simulink model "lab01"  (R2018a)
settings: Solver=VariableStepAuto  StartTime=0.0  StopTime=10.0  RelTol=1e-3
values from neighbouring files (symbols this model uses):
  dt = 5e-3    (= 0.005)    [lab0.m]    (also in lab0_step.m)
libraries: legoev3lib x4
settings Model: Creator=jacobdelrosario  LastModifiedBy=jacobdelrosario

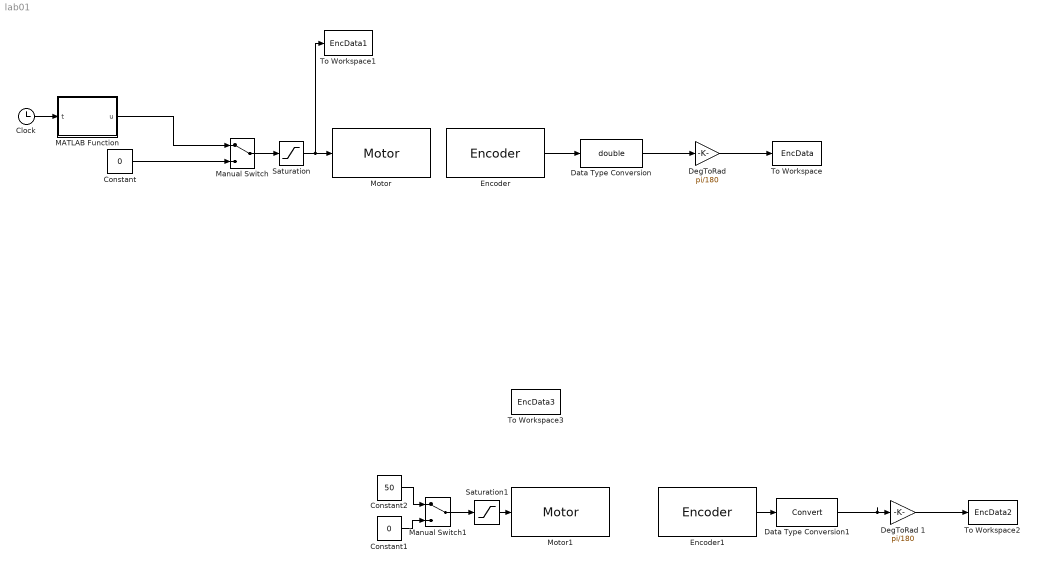
== system lab01 ==
  Clock : Clock
  Constant : Constant  Value=0  SampleTime=dt
  Constant1 : Constant  Value=0  SampleTime=dt
  Constant2 : Constant  Value=50  SampleTime=dt
  Data Type Conversion : DataTypeConversion  OutDataTypeStr=double
  Data Type Conversion1 : DataTypeConversion
  "DegToRad " : Gain  Gain=pi/180
  DegToRad 1 : Gain  Gain=pi/180
  Encoder : legoev3lib/Encoder  portNumber=A  opMode=No reset  sampleTime=dt
      settings: SourceProductName=Simulink Support Package for LEGO MINDSTORMS EV3 Hardware  SourceProductBaseCode=LEGOEV3
  Encoder1 : legoev3lib/Encoder  portNumber=A  opMode=Reset by external signal  sampleTime=dt
      settings: SourceProductName=Simulink Support Package for LEGO MINDSTORMS EV3 Hardware  SourceProductBaseCode=LEGOEV3
  MATLAB Function : MATLAB Function  TreatAsAtomicUnit=on
  Manual Switch : ManualSwitch
  Manual Switch1 : ManualSwitch
  Motor : legoev3lib/Motor  sportNumber=A  sstopAction=Brake
  Motor1 : legoev3lib/Motor  sportNumber=A  sstopAction=Brake
  Saturation : Saturate  UpperLimit=100  LowerLimit=-100
  Saturation1 : Saturate  UpperLimit=100  LowerLimit=-100
  To Workspace : ToWorkspace  VariableName=EncData  SaveFormat=Structure With Time  SampleTime=dt
  To Workspace1 : ToWorkspace  VariableName=EncData1  SaveFormat=Structure With Time  SampleTime=dt
  To Workspace2 : ToWorkspace  VariableName=EncData2  SaveFormat=Structure With Time  SampleTime=dt
  To Workspace3 : ToWorkspace  VariableName=EncData3  SaveFormat=Structure With Time  SampleTime=dt
  wires:
  Constant/1 -> Manual Switch/2
  Data Type Conversion/1 -> "DegToRad "/1
  Saturation/1 -> To Workspace1/1, Motor/1
  Encoder/1 -> Data Type Conversion/1
  Manual Switch/1 -> Saturation/1
  "DegToRad "/1 -> To Workspace/1
  Clock/1 -> MATLAB Function/1(t)
  MATLAB Function/1(u) -> Manual Switch/1
  Manual Switch1/1 -> Saturation1/1
  Encoder1/1 -> Data Type Conversion1/1
  Constant2/1 -> Manual Switch1/1
  Constant1/1 -> Manual Switch1/2
  Data Type Conversion1/1 -> DegToRad 1/1
  DegToRad 1/1 -> To Workspace2/1
  Saturation1/1 -> Motor1/1

== matlab function lab01/MATLAB Function ==
  data: t input; u output

function u = fcn(t)

if (t>2)
    u = 100;
else
    u = 0;
end


end
